simulink model "ctrl_HSMBObserver"  (R2015a)
settings: Solver=ode3  StartTime=0.0  StopTime=inf  FixedStep=0.01  RelTol=1e-3
values from neighbouring files (symbols this model uses):
  C = [C1;C2;C3;C4;C5;C6]    [initfile.m]    (also in thrustallocationQuadraticFixed.m)
  D = 3.0/100    (= 0.03)    [initfile.m]    (also in thrustallocationQuadraticFixed.m = 0.0411111111111)
  eps_c = 5    [initfile.m]
  epsilon = 0.5    [initfile.m]    (also in thrustallocationPseudo.m = u(10); thrustallocationQuadraticFixed.m = u(10))
  hd = c2d(H1,0.01,'foh')    [initfile.m]
  hd2 = c2d(H2,0.01,'zoh')    [initfile.m]
  I_s = 25000 /747225    (= 0.0334571246947)    [initfile.m]
  k_cc = 1    [initfile.m]
  K_omega = 0.3    [initfile.m]
  K_q1f = 0.0113    [initfile.m]
  K_q1r = K_q1f    (= 0.0113)    [initfile.m]
  K_q2f = 0.0117    [initfile.m]
  K_q2r = K_q2f    (= 0.0117)    [initfile.m]
  K_q3f = 0.0113    [initfile.m]
  K_q3r = K_q3f    (= 0.0113)    [initfile.m]
  K_q4f = 0.0169    [initfile.m]
  K_q4r = K_q4f    (= 0.0169)    [initfile.m]
  K_q5f = 0.0144    [initfile.m]
  K_q5r = K_q5f    (= 0.0144)    [initfile.m]
  K_q6f = 0.0168    [initfile.m]
  K_q6r = K_q6f    (= 0.0168)    [initfile.m]
  K_T1f = 0.3763    [initfile.m]
  K_T1r = K_T1f    (= 0.3763)    [initfile.m]
  K_T2f = 0.3901    [initfile.m]
  K_T2r = K_T2f    (= 0.3901)    [initfile.m]
  K_T3f = 0.3776    [initfile.m]
  K_T3r = K_T3f    (= 0.3776)    [initfile.m]
  K_T4f = 0.5641    [initfile.m]
  K_T4r = K_T4f    (= 0.5641)    [initfile.m]
  K_T5f = 0.4799    [initfile.m]
  K_T5r = K_T5f    (= 0.4799)    [initfile.m]
  K_T6f = 0.5588    [initfile.m]
  K_T6r = K_T6f    (= 0.5588)    [initfile.m]
  Kp = 3.3    [initfile.m]
  Max_Acceleration = 5    [initfile.m]
  Max_rotation = 12*sqrt(lambda)    [initfile.m]
  Max_thrust = 1.5    [initfile.m]
  Min_thrust = -0.8    [initfile.m]
  n_c = 5    [initfile.m]
  n_max = 152    [initfile.m]
  p_cc = 0.5    [initfile.m]
  pwm_thr1_backward = coeffvalues(ForceToPWM)    [initfile.m]
  pwm_thr1_forward = coeffvalues(ForceToPWM)    [initfile.m]
  pwm_thr2_backward = coeffvalues(ForceToPWM)    [initfile.m]
  pwm_thr2_forward = coeffvalues(ForceToPWM)    [initfile.m]
  pwm_thr3_backward = coeffvalues(ForceToPWM)    [initfile.m]
  pwm_thr3_forward = coeffvalues(ForceToPWM)    [initfile.m]
  pwm_thr4_backward = coeffvalues(ForceToPWM)    [initfile.m]
  pwm_thr4_forward = coeffvalues(ForceToPWM)    [initfile.m]
  pwm_thr5_backward = coeffvalues(ForceToPWM)    [initfile.m]
  pwm_thr5_forward = coeffvalues(ForceToPWM)    [initfile.m]
  pwm_thr6_backward = coeffvalues(ForceToPWM)    [initfile.m]
  pwm_thr6_forward = coeffvalues(ForceToPWM)    [initfile.m]
  Q_f0 = 0.3    [initfile.m]
  r_cc = 4    [initfile.m]
  Rho = Rho_m    (= 1000)    [initfile.m]
  ts = [-1 0]    [thrustallocationPseudo.m]    (also in thrustallocationQuadraticFixed.m)
undefined symbols (not defined in the file or in its folder): AFB, arm, Att, Control, Damping, FaultDet, Glob, Grip, IntActionType, Mass, NPO, Obs, Omg0_min, Q_max, ReferenceMdl, Sensor, Sim, SwLogic, tau, Thruster, Thruster_lock
libraries: dspmtrx3 x14, marine_gnc x11, simulink_extras x9, dspstat3 x9, simulink x9, dsparch4 x6, dspspect3 x6
(part 6 of 7)

== system ctrl_HSMBObserver/Thruster control /Thruster 6/Thruster control ==
  note: Q_ci
  note: Q_if
  note: Q_ff
  note: Q_ff0
  note: Q_ff1
  note: Friction compensation
  "T_d " : Inport
  n : Inport  Port=2
  Acceleration limiter : RateLimiter  RisingSlewLimit=Max_Acceleration  FallingSlewLimit=-Max_Acceleration  SampleTimeMode=inherited
  Constant1 : Constant  Value=hd.num{1,1}  VectorParams1D=off
  Constant2 : Constant  Value=hd.den{1,1}  VectorParams1D=off
  Controller chosen : MultiPortSwitch  Inputs=5
  Core controller : Subsystem
  Delay : Delay  DelayLength=1  InitialCondition=0
  Discrete Transfer Fcn : DiscreteTransferFcn  NumeratorSource=Input port  Numerator=[8.76e-05 0.0003481 8.648e-05]  DenominatorSource=Input port  Denominator=[1 -1.974 0.9746]  SampleTime=0.01  a0EqualsOne=on
      settings: InputPortMap=u0,p1,p3
  Discrete Derivative : simulink/Discrete/Discrete Derivative  gainval=1.0  ICPrevScaledInput=0.0  InputProcessing=Inherited  OutMin=[]  OutMax=[]  OutDataType=fixdt(1, 16)  OutScaling=2^-10  DoSatur=off
  Inertia compensation : Gain  Gain=I_s*2*pi
  MATLAB Function : MATLAB Function  TreatAsAtomicUnit=on
  Memory : Memory  X0=1
  NaN : Constant  Value=0
  Qf_0 : Gain  Gain=Q_f0
  Qff_0(nr) : Gain  Gain=epsilon/n_max
  Qff_1(nr) : Gain  Gain=K_omega*2*pi
  Sum : Sum  Inputs=+++
  Sum1 : Sum  Inputs=++|
  Supervisor : MATLAB Function  TreatAsAtomicUnit=on
  Trigonometric Function : Trigonometry  Operator=tanh
  Qc : Outport
  wires:
  Sum/1 -> Qc/1
  MATLAB Function/2(T_r) -> Core controller/2("Tr ")
  Discrete Derivative/1 -> Acceleration limiter/1
  Qff_0(nr)/1 -> Trigonometric Function/1
  Trigonometric Function/1 -> Qf_0/1
  Sum1/1 -> Sum/2
  Core controller/1(Q_cn) -> Controller chosen/2
  Core controller/4(Qcc) -> Controller chosen/5
  NaN/1 -> Controller chosen/6
  Memory/1 -> Supervisor/1(control), Controller chosen/1
  Qff_1(nr)/1 -> Sum1/2
  Qf_0/1 -> Sum1/1
  Controller chosen/1 -> Sum/3
  Inertia compensation/1 -> Sum/1
  Core controller/3(Qcp) -> Controller chosen/4
  Core controller/2(Qcq) -> Controller chosen/3
  [controller] -> Supervisor/2(input)
  "T_d "/1 -> MATLAB Function/1(Td)
  [Rho] -> MATLAB Function/4(rho)
  [D] -> MATLAB Function/5(D)
  [eps_c] -> MATLAB Function/6(eps_c)
  [n_c] -> MATLAB Function/7(n_c)
  Constant1/1 -> Discrete Transfer Fcn/2
  Constant2/1 -> Discrete Transfer Fcn/3
  MATLAB Function/1(n_d) -> Discrete Transfer Fcn/1
  n/1 -> Supervisor/3(n), Core controller/3("n ")
  Discrete Transfer Fcn/1 -> Discrete Derivative/1, Core controller/1(n_r), Delay/1, Qff_0(nr)/1, Qff_1(nr)/1
  Acceleration limiter/1 -> Inertia compensation/1
  Supervisor/1(u) -> Memory/1
  Delay/1 -> MATLAB Function/8(n_r)
  [Kt6r] -> MATLAB Function/3(K_t0r)
  [Kt6f] -> MATLAB Function/2(K_t0)

== system ctrl_HSMBObserver/To meters and radians, noise and sampling/Sensor noise models/Compass measurement noise module ==
  Band-Limited White Noise : simulink/Sources/Band-Limited White Noise  Cov=0.4*1e-12  Ts=0.01  seed=[23341]
  Bias compass : Constant  Value=0
  Sum : Sum  Inputs=+|+  SaturateOnIntegerOverflow=on
  Psi_noised : Outport
  wires:
  Sum/1 -> Psi_noised/1
  Band-Limited White Noise/1 -> Sum/2
  Bias compass/1 -> Sum/1

== system ctrl_HSMBObserver/To meters and radians, noise and sampling/Sensor noise models/Position (x,y) GPS measurement noise module ==
  note: Ionosphere
  note: Troposphere
  Band-Limited White Noise : simulink/Sources/Band-Limited White Noise  Cov=[1e-7 1e-7]  Ts=0.01  seed=[23341]
  Band-Limited White Noise1 Thermal effects : simulink/Sources/Band-Limited White Noise  Cov=[Sensor.GPS.Pow_thermal]  Ts=0.01  seed=[23341]
  Bias atmosphere : Constant  Value=[Sensor.GPS.Bias_atm]
  Sum : Sum  Inputs=+++  SaturateOnIntegerOverflow=on
  noised_pos (x.y) : Outport
  wires:
  Bias atmosphere/1 -> Sum/1
  Band-Limited White Noise1 Thermal effects/1 -> Sum/3
  Sum/1 -> noised_pos (x.y)/1
  Band-Limited White Noise/1 -> Sum/2

== system ctrl_HSMBObserver/Hybrid Controller/Controllers/Subsystem1/fault, update to q == 1 ==
  u_PD : Inport
  Action Port : ActionPort  ActionType=then
  u_PD_hold : Outport
  wires:
  u_PD/1 -> u_PD_hold/1

== system ctrl_HSMBObserver/Hybrid Controller/Controllers/Tau PD-control/GNC: "Transposed rotation matrix yaw: RTz_psi" ==
  note: GNC: "Transposed
      | rotation matrix yaw"
  psi : Inport
  eta_tilde : Inport  Port=2  PortDimensions=3
  Fcn : Fcn  Expr=cos(u(1))*u(2)+sin(u(1))*u(3)
  Fcn1 : Fcn  Expr=-sin(u(1))*u(2)+cos(u(1))*u(3)
  Fcn2 : Fcn  Expr=u(4)
  Mux2 : Mux  Inputs=2
  Mux3 : Mux  Inputs=3
  R_T*eta_tilde : Outport
  wires:
  Mux2/1 -> Fcn1/1, Fcn/1, Fcn2/1
  Fcn/1 -> Mux3/1  "x_dot"
  Fcn1/1 -> Mux3/2  "y_dot"
  Fcn2/1 -> Mux3/3  "psi_dot"
  Mux3/1 -> R_T*eta_tilde/1  "eta_dot"
  psi/1 -> Mux2/1
  eta_tilde/1 -> Mux2/2

== system ctrl_HSMBObserver/Hybrid Controller/Controllers/Tau integral action: Normal or AFF/GNC: "Transposed rotation matrix yaw: RTz_psi"3 ==
  note: GNC: "Transposed
      | rotation matrix yaw"
  psi : Inport
  int_NED : Inport  Port=2  PortDimensions=3
  Fcn : Fcn  Expr=cos(u(1))*u(2)+sin(u(1))*u(3)
  Fcn1 : Fcn  Expr=-sin(u(1))*u(2)+cos(u(1))*u(3)
  Fcn2 : Fcn  Expr=u(4)
  Mux2 : Mux  Inputs=2
  Mux3 : Mux  Inputs=3
  R_T*eta_tilde : Outport
  wires:
  Mux2/1 -> Fcn1/1, Fcn/1, Fcn2/1
  Fcn/1 -> Mux3/1  "x_dot"
  Fcn1/1 -> Mux3/2  "y_dot"
  Fcn2/1 -> Mux3/3  "psi_dot"
  Mux3/1 -> R_T*eta_tilde/1  "eta_dot"
  psi/1 -> Mux2/1
  int_NED/1 -> Mux2/2

== system ctrl_HSMBObserver/Hybrid Controller/Controllers/Tau integral action: Normal or AFF/R(psi)nu1 ==
  Nu : Inport
  psi : Inport  Port=2
  Demux : Demux  Outputs=3
  Mux : Mux  Inputs=3
  Mux1 : Mux  Inputs=3
  Row1 : Fcn  Expr=cos(u(3))*u(1)-sin(u(3))*u(2)
  Row2 : Fcn  Expr=sin(u(3))*u(1)+cos(u(3))*u(2)
  Eta : Outport
  wires:
  Demux/3 -> Mux1/3
  Nu/1 -> Demux/1
  psi/1 -> Mux/3
  Demux/1 -> Mux/1
  Demux/2 -> Mux/2
  Mux/1 -> Row1/1, Row2/1
  Mux1/1 -> Eta/1
  Row2/1 -> Mux1/2
  Row1/1 -> Mux1/1

== system ctrl_HSMBObserver/Hybrid Controller/Nonlinear observer, version implemented 04.26.2016/Hybridgains - kappa determination/Subsystem ==
  eta_f : Inport
  Demux : Demux  Outputs=3
  Dot Product : DotProduct  InputSameDT=on  OutDataTypeStr=Inherit: Inherit via internal rule
  Mux : Mux  Inputs=3
  Radians to Degrees : simulink_extras/Transformations/Radians to Degrees
  Transpose : Math  Operator=transpose  SaturateOnIntegerOverflow=on
  norm(eta_eta_f) : Outport
  wires:
  Dot Product/1 -> norm(eta_eta_f)/1
  Demux/3 -> Radians to Degrees/1
  Demux/1 -> Mux/1
  Demux/2 -> Mux/2
  Radians to Degrees/1 -> Mux/3
  Mux/1 -> Transpose/1, Dot Product/2
  Transpose/1 -> Dot Product/1
  eta_f/1 -> Demux/1

== system ctrl_HSMBObserver/Hybrid Controller/Peak Frequency FFT/CalmWater choose PID1/If Action Subsystem ==
  Action Port : ActionPort  ActionType=then
  Constant : Constant  Value=Omg0_min
  omega_p : Outport
  wires:
  Constant/1 -> omega_p/1

== system ctrl_HSMBObserver/Hybrid Controller/Peak Frequency FFT/CalmWater choose PID1/If Action Subsystem1 ==
  In1 : Inport
  Action Port : ActionPort  ActionType=else
  Out1 : Outport
  wires:
  In1/1 -> Out1/1

== system ctrl_HSMBObserver/Hybrid Controller/Peak Frequency FFT/estimate w_p/Spectral Analysis ==
  eta_6DOF : Inport
  Analog Filter Design{,1..5} (6 alike) : dsparch4/Analog Filter Design  method=Butterworth  filttype=Highpass  N=2  Wlo=Control.SA.pssbnd  Whi=80  Rp=2  Rs=40
  Demux : Demux  Outputs=6
  FFT : Subsystem
  w_p : Outport
  wires:
  eta_6DOF/1 -> Demux/1
  Demux/1 -> Analog Filter Design/1
  Analog Filter Design/1 -> FFT/1(surge)
  Analog Filter Design1/1 -> FFT/2(sway)
  Analog Filter Design2/1 -> FFT/3(heave)
  FFT/1(w_p) -> w_p/1
  Demux/3 -> Analog Filter Design2/1
  Demux/2 -> Analog Filter Design1/1
  Demux/5 -> Analog Filter Design3/1
  Demux/6 -> Analog Filter Design4/1
  Analog Filter Design3/1 -> FFT/5(pitch)
  Analog Filter Design4/1 -> FFT/6(yaw)
  Demux/4 -> Analog Filter Design5/1
  Analog Filter Design5/1 -> FFT/4(roll)

== system ctrl_HSMBObserver/Hybrid Controller/Switching logic/Desired yaw rate/Stay with the current controlller ==
  In1 : Inport
  Action Port : ActionPort  ActionType=else
  Out1 : Outport
  wires:
  In1/1 -> Out1/1

== system ctrl_HSMBObserver/Hybrid Controller/Switching logic/Desired yaw rate/Switch to grip ==
  Action Port : ActionPort  ActionType=then
  Constant : Constant  Value=2
  Out1 : Outport
  wires:
  Constant/1 -> Out1/1

== system ctrl_HSMBObserver/Hybrid Controller/Switching logic/Performance/Stay with the current controlller ==
  In1 : Inport
  Action Port : ActionPort  ActionType=else
  Out1 : Outport
  wires:
  In1/1 -> Out1/1

== system ctrl_HSMBObserver/Hybrid Controller/Switching logic/Performance/Switch to NPO ==
  Action Port : ActionPort  ActionType=then
  Constant : Constant
  Out1 : Outport
  wires:
  Constant/1 -> Out1/1

== system ctrl_HSMBObserver/Hybrid Controller/Switching logic/Performance/Switch to grip ==
  Action Port : ActionPort  ActionType=elseif
  Constant : Constant  Value=2
  Out1 : Outport
  wires:
  Constant/1 -> Out1/1

== system ctrl_HSMBObserver/Hybrid Controller/nPDF/Subsystem/R^TKdR ==
  eta : Inport
  nu : Inport  Port=2
  Kd : Inport  Port=3
  Create Diagonal Matrix3 : dspmtrx3/Create Diagonal Matrix
  Matrix Multiply3 : Product  Multiplication=Matrix(*)
  Rotation matrix in yaw 1 : marine_gnc/Models/ Kinematics/Rotation matrix in yaw 
  Selector : Selector  InputPortWidth=3  Indices=3
  Transposed rotation matrix in yaw1 : marine_gnc/Models/ Kinematics/Transposed rotation  matrix in yaw
  R^TKdR*nu : Outport
  wires:
  Selector/1 -> Rotation matrix in yaw 1/1, Transposed rotation matrix in yaw1/1
  eta/1 -> Selector/1
  nu/1 -> Rotation matrix in yaw 1/2
  Transposed rotation matrix in yaw1/1 -> R^TKdR*nu/1
  Rotation matrix in yaw 1/1 -> Matrix Multiply3/2
  Create Diagonal Matrix3/1 -> Matrix Multiply3/1
  Kd/1 -> Create Diagonal Matrix3/1
  Matrix Multiply3/1 -> Transposed rotation matrix in yaw1/2

== system ctrl_HSMBObserver/Hybrid Controller/nPDF/Subsystem/S(r)*nu ==
  nu : Inport
  Constant : Constant  Value=[0 -1 0;1 0 0;0 0 0]
  Product : Product  Multiplication=Matrix(*)
  Product1 : Product
  Selector1 : Selector  InputPortWidth=3  Indices=3
  S(r)*nu : Outport
  wires:
  Product/1 -> S(r)*nu/1
  Product1/1 -> Product/1
  nu/1 -> Product/2, Selector1/1
  Constant/1 -> Product1/2
  Selector1/1 -> Product1/1

== system ctrl_HSMBObserver/Thruster control /Thruster 1/Thruster control/Core controller ==
  note: Core controller: Shaft speed
  n_r : Inport
  "Tr " : Inport  Port=2
  "n " : Inport  Port=3
  Core controller: Torque,Power and Combined Torque/Power : MATLAB Function  TreatAsAtomicUnit=on
  Integrator : Integrator  ExternalReset=either  UpperSaturationLimit=Q_max  LowerSaturationLimit=-Q_max
  Ki : Gain  Gain=Kp/0.05
  Kp : Gain  Gain=Kp
  Sum : Sum  Inputs=+|-
  Sum1 : Sum  Inputs=|++
  reset : S-Function  Priority=1  FunctionName=NIVeriStandIO  Parameters=width dtype portnum stime stype btype  mask(NI VeriStand Inport){portnum=1, width=-1, stime=-1, dtype=auto, stype=auto, btype=1}
      mask prompts: portnum "Port number:"; width "Port dimensions (-1 for dynamically sized):"; stime "Sample time (-1 for inherited):"; dtype "Data type:"; stype "Signal type:"; btype "Block type:"
      mask help: Use this inport on any level of nested subsystems to allow NI VeriStand software to map signals to it.
      mask init:
      | NIVeriStandIO_init;
      settings: CopyFcn=NIVeriStand_MDL_functions('', 'IO_copy');  DeleteFcn=NIVeriStand_MDL_functions('', 'IO_delete');  MoveFcn=set_param(gcb, 'Mask', 'on');
      mask Callback portnum: NIVeriStand_MDL_functions('', 'IO_setportnum');
      mask TypeOptions dtype: auto | double | single | int8 | uint8 | int16 | uint16 | int32 | uint32 | boolean
      mask Callback dtype: NIVeriStand_MDL_functions('', 'IO_booleansignal');
      mask TypeOptions stype: auto | real | complex
      mask Display:
      | patch([-x x], [-y y], [.90980 .81960 .32156]);
      | plot([xrad -x x xrad], [yrad -y y yrad]);
      | fprintf('NI In%d', portnum);
  Q_cn : Outport
  Qcq : Outport  Port=2
  Qcp : Outport  Port=3
  Qcc : Outport  Port=4
  wires:
  [k_cc] -> Core controller: Torque,Power and Combined Torque/Power/1(k_cc)
  [p_cc] -> Core controller: Torque,Power and Combined Torque/Power/2(p_cc)
  [r_cc] -> Core controller: Torque,Power and Combined Torque/Power/3(r_cc)
  Core controller: Torque,Power and Combined Torque/Power/3(Qcc) -> Qcc/1
  [Kt1f] -> Core controller: Torque,Power and Combined Torque/Power/5(K_t0)
  [D] -> Core controller: Torque,Power and Combined Torque/Power/7(D)
  [Kq1f] -> Core controller: Torque,Power and Combined Torque/Power/6(K_q0)
  [Rho] -> Core controller: Torque,Power and Combined Torque/Power/9(rho)
  "n "/1 -> Sum/2, Core controller: Torque,Power and Combined Torque/Power/4(n)
  "Tr "/1 -> Core controller: Torque,Power and Combined Torque/Power/8(Tr)
  Core controller: Torque,Power and Combined Torque/Power/2(Qcp) -> Qcp/1
  Core controller: Torque,Power and Combined Torque/Power/1(Qcq) -> Qcq/1
  n_r/1 -> Sum/1
  Ki/1 -> Integrator/1
  Kp/1 -> Sum1/1
  Integrator/1 -> Sum1/2
  Sum1/1 -> Q_cn/1
  Sum/1 -> Ki/1, Kp/1
  reset/1 -> Integrator/2
  [eps_c] -> Core controller: Torque,Power and Combined Torque/Power/10(eps_c)
  [Kt1r] -> Core controller: Torque,Power and Combined Torque/Power/11(K_t0r)
  [Kq1r] -> Core controller: Torque,Power and Combined Torque/Power/12(K_q0r)

== system ctrl_HSMBObserver/Thruster control /Thruster 2/Thruster control/Core controller ==
  note: Core controller: Shaft speed
  n_r : Inport
  "Tr " : Inport  Port=2
  "n " : Inport  Port=3
  Core controller: Torque,Power and Combined Torque/Power : MATLAB Function  TreatAsAtomicUnit=on
  Integrator : Integrator  ExternalReset=either  UpperSaturationLimit=Q_max  LowerSaturationLimit=-Q_max
  Ki : Gain  Gain=Kp/0.05
  Kp : Gain  Gain=Kp
  Sum : Sum  Inputs=+|-
  Sum1 : Sum  Inputs=|++
  reset : S-Function  Priority=1  FunctionName=NIVeriStandIO  Parameters=width dtype portnum stime stype btype  mask(NI VeriStand Inport){portnum=1, width=-1, stime=-1, dtype=auto, stype=auto, btype=1}
      mask prompts: portnum "Port number:"; width "Port dimensions (-1 for dynamically sized):"; stime "Sample time (-1 for inherited):"; dtype "Data type:"; stype "Signal type:"; btype "Block type:"
      mask help: Use this inport on any level of nested subsystems to allow NI VeriStand software to map signals to it.
      mask init:
      | NIVeriStandIO_init;
      settings: CopyFcn=NIVeriStand_MDL_functions('', 'IO_copy');  DeleteFcn=NIVeriStand_MDL_functions('', 'IO_delete');  MoveFcn=set_param(gcb, 'Mask', 'on');
      mask Callback portnum: NIVeriStand_MDL_functions('', 'IO_setportnum');
      mask TypeOptions dtype: auto | double | single | int8 | uint8 | int16 | uint16 | int32 | uint32 | boolean
      mask Callback dtype: NIVeriStand_MDL_functions('', 'IO_booleansignal');
      mask TypeOptions stype: auto | real | complex
      mask Display:
      | patch([-x x], [-y y], [.90980 .81960 .32156]);
      | plot([xrad -x x xrad], [yrad -y y yrad]);
      | fprintf('NI In%d', portnum);
  Q_cn : Outport
  Qcq : Outport  Port=2
  Qcp : Outport  Port=3
  Qcc : Outport  Port=4
  wires:
  n_r/1 -> Sum/1
  Ki/1 -> Integrator/1
  Kp/1 -> Sum1/1
  Integrator/1 -> Sum1/2
  Sum/1 -> Ki/1, Kp/1
  Sum1/1 -> Q_cn/1
  reset/1 -> Integrator/2
  [k_cc] -> Core controller: Torque,Power and Combined Torque/Power/1(k_cc)
  [p_cc] -> Core controller: Torque,Power and Combined Torque/Power/2(p_cc)
  [r_cc] -> Core controller: Torque,Power and Combined Torque/Power/3(r_cc)
  Core controller: Torque,Power and Combined Torque/Power/3(Qcc) -> Qcc/1
  [Kt2f] -> Core controller: Torque,Power and Combined Torque/Power/5(K_t0)
  [D] -> Core controller: Torque,Power and Combined Torque/Power/7(D)
  [Kq2f] -> Core controller: Torque,Power and Combined Torque/Power/6(K_q0)
  [Rho] -> Core controller: Torque,Power and Combined Torque/Power/9(rho)
  "n "/1 -> Core controller: Torque,Power and Combined Torque/Power/4(n), Sum/2
  "Tr "/1 -> Core controller: Torque,Power and Combined Torque/Power/8(Tr)
  Core controller: Torque,Power and Combined Torque/Power/2(Qcp) -> Qcp/1
  Core controller: Torque,Power and Combined Torque/Power/1(Qcq) -> Qcq/1
  [eps_c] -> Core controller: Torque,Power and Combined Torque/Power/10(eps_c)
  [Kt2r] -> Core controller: Torque,Power and Combined Torque/Power/11(K_t0r)
  [Kq2r] -> Core controller: Torque,Power and Combined Torque/Power/12(K_q0r)

== system ctrl_HSMBObserver/Thruster control /Thruster 3/Thruster control/Core controller ==
  note: Core controller: Shaft speed
  n_r : Inport
  "Tr " : Inport  Port=2
  "n " : Inport  Port=3
  Core controller: Torque,Power and Combined Torque/Power : MATLAB Function  TreatAsAtomicUnit=on
  Integrator : Integrator  ExternalReset=either  UpperSaturationLimit=Q_max  LowerSaturationLimit=-Q_max
  Ki : Gain  Gain=Kp/0.05
  Kp : Gain  Gain=Kp
  Sum : Sum  Inputs=+|-
  Sum1 : Sum  Inputs=|++
  reset : S-Function  Priority=1  FunctionName=NIVeriStandIO  Parameters=width dtype portnum stime stype btype  mask(NI VeriStand Inport){portnum=1, width=-1, stime=-1, dtype=auto, stype=auto, btype=1}
      mask prompts: portnum "Port number:"; width "Port dimensions (-1 for dynamically sized):"; stime "Sample time (-1 for inherited):"; dtype "Data type:"; stype "Signal type:"; btype "Block type:"
      mask help: Use this inport on any level of nested subsystems to allow NI VeriStand software to map signals to it.
      mask init:
      | NIVeriStandIO_init;
      settings: CopyFcn=NIVeriStand_MDL_functions('', 'IO_copy');  DeleteFcn=NIVeriStand_MDL_functions('', 'IO_delete');  MoveFcn=set_param(gcb, 'Mask', 'on');
      mask Callback portnum: NIVeriStand_MDL_functions('', 'IO_setportnum');
      mask TypeOptions dtype: auto | double | single | int8 | uint8 | int16 | uint16 | int32 | uint32 | boolean
      mask Callback dtype: NIVeriStand_MDL_functions('', 'IO_booleansignal');
      mask TypeOptions stype: auto | real | complex
      mask Display:
      | patch([-x x], [-y y], [.90980 .81960 .32156]);
      | plot([xrad -x x xrad], [yrad -y y yrad]);
      | fprintf('NI In%d', portnum);
  Q_cn : Outport
  Qcq : Outport  Port=2
  Qcp : Outport  Port=3
  Qcc : Outport  Port=4
  wires:
  n_r/1 -> Sum/1
  Ki/1 -> Integrator/1
  Kp/1 -> Sum1/1
  Integrator/1 -> Sum1/2
  Sum/1 -> Ki/1, Kp/1
  Sum1/1 -> Q_cn/1
  reset/1 -> Integrator/2
  [k_cc] -> Core controller: Torque,Power and Combined Torque/Power/1(k_cc)
  [p_cc] -> Core controller: Torque,Power and Combined Torque/Power/2(p_cc)
  [r_cc] -> Core controller: Torque,Power and Combined Torque/Power/3(r_cc)
  Core controller: Torque,Power and Combined Torque/Power/3(Qcc) -> Qcc/1
  [Kt3f] -> Core controller: Torque,Power and Combined Torque/Power/5(K_t0)
  [D] -> Core controller: Torque,Power and Combined Torque/Power/7(D)
  [Kq3f] -> Core controller: Torque,Power and Combined Torque/Power/6(K_q0)
  [Rho] -> Core controller: Torque,Power and Combined Torque/Power/9(rho)
  "n "/1 -> Sum/2, Core controller: Torque,Power and Combined Torque/Power/4(n)
  "Tr "/1 -> Core controller: Torque,Power and Combined Torque/Power/8(Tr)
  Core controller: Torque,Power and Combined Torque/Power/2(Qcp) -> Qcp/1
  Core controller: Torque,Power and Combined Torque/Power/1(Qcq) -> Qcq/1
  [eps_c] -> Core controller: Torque,Power and Combined Torque/Power/10(eps_c)
  [Kt3r] -> Core controller: Torque,Power and Combined Torque/Power/11(K_t0r)
  [Kq3r] -> Core controller: Torque,Power and Combined Torque/Power/12(K_q0r)

== system ctrl_HSMBObserver/Thruster control /Thruster 4/Thruster control/Core controller ==
  note: Core controller: Shaft speed
  n_r : Inport
  "Tr " : Inport  Port=2
  "n " : Inport  Port=3
  Core controller: Torque,Power and Combined Torque/Power : MATLAB Function  TreatAsAtomicUnit=on
  Integrator : Integrator  ExternalReset=either  UpperSaturationLimit=Q_max  LowerSaturationLimit=-Q_max
  Ki : Gain  Gain=Kp/0.05
  Kp : Gain  Gain=Kp
  Sum : Sum  Inputs=+|-
  Sum1 : Sum  Inputs=|++
  reset : S-Function  Priority=1  FunctionName=NIVeriStandIO  Parameters=width dtype portnum stime stype btype  mask(NI VeriStand Inport){portnum=1, width=-1, stime=-1, dtype=auto, stype=auto, btype=1}
      mask prompts: portnum "Port number:"; width "Port dimensions (-1 for dynamically sized):"; stime "Sample time (-1 for inherited):"; dtype "Data type:"; stype "Signal type:"; btype "Block type:"
      mask help: Use this inport on any level of nested subsystems to allow NI VeriStand software to map signals to it.
      mask init:
      | NIVeriStandIO_init;
      settings: CopyFcn=NIVeriStand_MDL_functions('', 'IO_copy');  DeleteFcn=NIVeriStand_MDL_functions('', 'IO_delete');  MoveFcn=set_param(gcb, 'Mask', 'on');
      mask Callback portnum: NIVeriStand_MDL_functions('', 'IO_setportnum');
      mask TypeOptions dtype: auto | double | single | int8 | uint8 | int16 | uint16 | int32 | uint32 | boolean
      mask Callback dtype: NIVeriStand_MDL_functions('', 'IO_booleansignal');
      mask TypeOptions stype: auto | real | complex
      mask Display:
      | patch([-x x], [-y y], [.90980 .81960 .32156]);
      | plot([xrad -x x xrad], [yrad -y y yrad]);
      | fprintf('NI In%d', portnum);
  Q_cn : Outport
  Qcq : Outport  Port=2
  Qcp : Outport  Port=3
  Qcc : Outport  Port=4
  wires:
  n_r/1 -> Sum/1
  Ki/1 -> Integrator/1
  Kp/1 -> Sum1/1
  Integrator/1 -> Sum1/2
  Sum/1 -> Ki/1, Kp/1
  Sum1/1 -> Q_cn/1
  [k_cc] -> Core controller: Torque,Power and Combined Torque/Power/1(k_cc)
  [p_cc] -> Core controller: Torque,Power and Combined Torque/Power/2(p_cc)
  [r_cc] -> Core controller: Torque,Power and Combined Torque/Power/3(r_cc)
  Core controller: Torque,Power and Combined Torque/Power/3(Qcc) -> Qcc/1
  [Kt4f] -> Core controller: Torque,Power and Combined Torque/Power/5(K_t0)
  [D] -> Core controller: Torque,Power and Combined Torque/Power/7(D)
  [Kq4f] -> Core controller: Torque,Power and Combined Torque/Power/6(K_q0)
  [Rho] -> Core controller: Torque,Power and Combined Torque/Power/9(rho)
  "n "/1 -> Core controller: Torque,Power and Combined Torque/Power/4(n), Sum/2
  "Tr "/1 -> Core controller: Torque,Power and Combined Torque/Power/8(Tr)
  Core controller: Torque,Power and Combined Torque/Power/2(Qcp) -> Qcp/1
  Core controller: Torque,Power and Combined Torque/Power/1(Qcq) -> Qcq/1
  [eps_c] -> Core controller: Torque,Power and Combined Torque/Power/10(eps_c)
  [Kt4r] -> Core controller: Torque,Power and Combined Torque/Power/11(K_t0r)
  [Kq4r] -> Core controller: Torque,Power and Combined Torque/Power/12(K_q0r)
  reset/1 -> Integrator/2

== system ctrl_HSMBObserver/Thruster control /Thruster 5/Thruster control/Core controller ==
  note: Core controller: Shaft speed
  n_r : Inport
  "Tr " : Inport  Port=2
  "n " : Inport  Port=3
  Core controller: Torque,Power and Combined Torque/Power : MATLAB Function  TreatAsAtomicUnit=on
  Integrator : Integrator  ExternalReset=either  UpperSaturationLimit=Q_max  LowerSaturationLimit=-Q_max
  Ki : Gain  Gain=Kp/0.05
  Kp : Gain  Gain=Kp
  Sum : Sum  Inputs=+|-
  Sum1 : Sum  Inputs=|++
  reset : S-Function  Priority=1  FunctionName=NIVeriStandIO  Parameters=width dtype portnum stime stype btype  mask(NI VeriStand Inport){portnum=1, width=-1, stime=-1, dtype=auto, stype=auto, btype=1}
      mask prompts: portnum "Port number:"; width "Port dimensions (-1 for dynamically sized):"; stime "Sample time (-1 for inherited):"; dtype "Data type:"; stype "Signal type:"; btype "Block type:"
      mask help: Use this inport on any level of nested subsystems to allow NI VeriStand software to map signals to it.
      mask init:
      | NIVeriStandIO_init;
      settings: CopyFcn=NIVeriStand_MDL_functions('', 'IO_copy');  DeleteFcn=NIVeriStand_MDL_functions('', 'IO_delete');  MoveFcn=set_param(gcb, 'Mask', 'on');
      mask Callback portnum: NIVeriStand_MDL_functions('', 'IO_setportnum');
      mask TypeOptions dtype: auto | double | single | int8 | uint8 | int16 | uint16 | int32 | uint32 | boolean
      mask Callback dtype: NIVeriStand_MDL_functions('', 'IO_booleansignal');
      mask TypeOptions stype: auto | real | complex
      mask Display:
      | patch([-x x], [-y y], [.90980 .81960 .32156]);
      | plot([xrad -x x xrad], [yrad -y y yrad]);
      | fprintf('NI In%d', portnum);
  Q_cn : Outport
  Qcq : Outport  Port=2
  Qcp : Outport  Port=3
  Qcc : Outport  Port=4
  wires:
  n_r/1 -> Sum/1
  Ki/1 -> Integrator/1
  Kp/1 -> Sum1/1
  Integrator/1 -> Sum1/2
  Sum/1 -> Ki/1, Kp/1
  Sum1/1 -> Q_cn/1
  reset/1 -> Integrator/2
  [k_cc] -> Core controller: Torque,Power and Combined Torque/Power/1(k_cc)
  [p_cc] -> Core controller: Torque,Power and Combined Torque/Power/2(p_cc)
  [r_cc] -> Core controller: Torque,Power and Combined Torque/Power/3(r_cc)
  Core controller: Torque,Power and Combined Torque/Power/3(Qcc) -> Qcc/1
  [Kt5f] -> Core controller: Torque,Power and Combined Torque/Power/5(K_t0)
  [D] -> Core controller: Torque,Power and Combined Torque/Power/7(D)
  [Kq5f] -> Core controller: Torque,Power and Combined Torque/Power/6(K_q0)
  [Rho] -> Core controller: Torque,Power and Combined Torque/Power/9(rho)
  "n "/1 -> Core controller: Torque,Power and Combined Torque/Power/4(n), Sum/2
  "Tr "/1 -> Core controller: Torque,Power and Combined Torque/Power/8(Tr)
  Core controller: Torque,Power and Combined Torque/Power/2(Qcp) -> Qcp/1
  Core controller: Torque,Power and Combined Torque/Power/1(Qcq) -> Qcq/1
  [eps_c] -> Core controller: Torque,Power and Combined Torque/Power/10(eps_c)
  [Kt5r] -> Core controller: Torque,Power and Combined Torque/Power/11(K_t0r)
  [Kq5r] -> Core controller: Torque,Power and Combined Torque/Power/12(K_q0r)

== system ctrl_HSMBObserver/Thruster control /Thruster 6/Thruster control/Core controller ==
  note: Core controller: Shaft speed
  n_r : Inport
  "Tr " : Inport  Port=2
  "n " : Inport  Port=3
  Core controller: Torque,Power and Combined Torque/Power : MATLAB Function  TreatAsAtomicUnit=on
  Integrator : Integrator  ExternalReset=either  UpperSaturationLimit=Q_max  LowerSaturationLimit=-Q_max
  Ki : Gain  Gain=Kp/0.05
  Kp : Gain  Gain=Kp
  Sum : Sum  Inputs=+|-
  Sum1 : Sum  Inputs=|++
  reset : S-Function  Priority=1  FunctionName=NIVeriStandIO  Parameters=width dtype portnum stime stype btype  mask(NI VeriStand Inport){portnum=1, width=-1, stime=-1, dtype=auto, stype=auto, btype=1}
      mask prompts: portnum "Port number:"; width "Port dimensions (-1 for dynamically sized):"; stime "Sample time (-1 for inherited):"; dtype "Data type:"; stype "Signal type:"; btype "Block type:"
      mask help: Use this inport on any level of nested subsystems to allow NI VeriStand software to map signals to it.
      mask init:
      | NIVeriStandIO_init;
      settings: CopyFcn=NIVeriStand_MDL_functions('', 'IO_copy');  DeleteFcn=NIVeriStand_MDL_functions('', 'IO_delete');  MoveFcn=set_param(gcb, 'Mask', 'on');
      mask Callback portnum: NIVeriStand_MDL_functions('', 'IO_setportnum');
      mask TypeOptions dtype: auto | double | single | int8 | uint8 | int16 | uint16 | int32 | uint32 | boolean
      mask Callback dtype: NIVeriStand_MDL_functions('', 'IO_booleansignal');
      mask TypeOptions stype: auto | real | complex
      mask Display:
      | patch([-x x], [-y y], [.90980 .81960 .32156]);
      | plot([xrad -x x xrad], [yrad -y y yrad]);
      | fprintf('NI In%d', portnum);
  Q_cn : Outport
  Qcq : Outport  Port=2
  Qcp : Outport  Port=3
  Qcc : Outport  Port=4
  wires:
  n_r/1 -> Sum/1
  Ki/1 -> Integrator/1
  Kp/1 -> Sum1/1
  Integrator/1 -> Sum1/2
  Sum/1 -> Ki/1, Kp/1
  Sum1/1 -> Q_cn/1
  reset/1 -> Integrator/2
  [k_cc] -> Core controller: Torque,Power and Combined Torque/Power/1(k_cc)
  [p_cc] -> Core controller: Torque,Power and Combined Torque/Power/2(p_cc)
  [r_cc] -> Core controller: Torque,Power and Combined Torque/Power/3(r_cc)
  Core controller: Torque,Power and Combined Torque/Power/3(Qcc) -> Qcc/1
  [Kt6f] -> Core controller: Torque,Power and Combined Torque/Power/5(K_t0)
  [D] -> Core controller: Torque,Power and Combined Torque/Power/7(D)
  [Kq6f] -> Core controller: Torque,Power and Combined Torque/Power/6(K_q0)
  [Rho] -> Core controller: Torque,Power and Combined Torque/Power/9(rho)
  "n "/1 -> Core controller: Torque,Power and Combined Torque/Power/4(n), Sum/2
  "Tr "/1 -> Core controller: Torque,Power and Combined Torque/Power/8(Tr)
  Core controller: Torque,Power and Combined Torque/Power/2(Qcp) -> Qcp/1
  Core controller: Torque,Power and Combined Torque/Power/1(Qcq) -> Qcq/1
  [eps_c] -> Core controller: Torque,Power and Combined Torque/Power/10(eps_c)
  [Kt6r] -> Core controller: Torque,Power and Combined Torque/Power/11(K_t0r)
  [Kq6r] -> Core controller: Torque,Power and Combined Torque/Power/12(K_q0r)

== system ctrl_HSMBObserver/Hybrid Controller/Peak Frequency FFT/estimate w_p/Spectral Analysis/FFT ==
  surge : Inport
  sway : Inport  Port=2
  heave : Inport  Port=3
  roll : Inport  Port=4
  pitch : Inport  Port=5
  yaw : Inport  Port=6
  Hz_to_rad/s : Gain  Gain=2*pi  SaturateOnIntegerOverflow=on  OutDataTypeStr=Inherit: Same as input  ParamDataTypeStr=Inherit: Same as input
  Rate Transition : RateTransition  OutPortSampleTime=0.01
  "wave freq estimator using the Burg parametric/ max entropy method " : Subsystem  mask{Fs=Control.SA.SampleFreq, b1=Control.SA.BufferSize, nfft=Control.SA.FFTlength, burg_order=Control.SA.BurgOrder, ovl=Control.SA.Overlap}
      mask prompts: Fs "Sample frequency=Fs"; b1 "Size buffer 1=b1"; nfft "FFT length=nfft"; burg_order "Order of Burg estim=burg_order"; ovl "Overlap=ovl"
  w_p : Outport
  wires:
  "wave freq estimator using the Burg parametric/ max entropy method "/1(w0_hat) -> Hz_to_rad/s/1
  surge/1 -> "wave freq estimator using the Burg parametric/ max entropy method "/1(x_pos)
  sway/1 -> "wave freq estimator using the Burg parametric/ max entropy method "/2(y_pos)
  heave/1 -> "wave freq estimator using the Burg parametric/ max entropy method "/3(z_pos)
  Hz_to_rad/s/1 -> Rate Transition/1
  roll/1 -> "wave freq estimator using the Burg parametric/ max entropy method "/4(phi_pos)
  pitch/1 -> "wave freq estimator using the Burg parametric/ max entropy method "/5(theta_pos)
  yaw/1 -> "wave freq estimator using the Burg parametric/ max entropy method "/6(psi_pos)
  Rate Transition/1 -> w_p/1

== system ctrl_HSMBObserver/Hybrid Controller/Peak Frequency FFT/estimate w_p/Spectral Analysis/FFT/wave freq estimator using the Burg parametric// max entropy method  ==
  x_pos : Inport
  y_pos : Inport  Port=2
  z_pos : Inport  Port=3
  phi_pos : Inport  Port=4
  theta_pos : Inport  Port=5
  psi_pos : Inport  Port=6
  PSD estimation with Burg method : Subsystem
  Peak frequency estimation : Subsystem
  w0_hat : Outport
  wires:
  PSD estimation with Burg method/1(x_PSD) -> Peak frequency estimation/1(x_PSD)
  PSD estimation with Burg method/2(y_PSD) -> Peak frequency estimation/2(y_PSD)
  PSD estimation with Burg method/3(z_PSD) -> Peak frequency estimation/3(z_PSD)
  PSD estimation with Burg method/4(phi_PSD) -> Peak frequency estimation/4(phi_PSD)
  PSD estimation with Burg method/5(theta_PSD) -> Peak frequency estimation/5(theta_PSD)
  PSD estimation with Burg method/6(psi_PSD) -> Peak frequency estimation/6(psi_PSD)
  x_pos/1 -> PSD estimation with Burg method/1(x_pos)
  y_pos/1 -> PSD estimation with Burg method/2(y_pos)
  z_pos/1 -> PSD estimation with Burg method/3(z_pos)
  phi_pos/1 -> PSD estimation with Burg method/4(phi_pos)
  theta_pos/1 -> PSD estimation with Burg method/5(theta_pos)
  psi_pos/1 -> PSD estimation with Burg method/6(psi_pos)
  Peak frequency estimation/1(w0_hat) -> w0_hat/1

== system ctrl_HSMBObserver/Hybrid Controller/Peak Frequency FFT/estimate w_p/Spectral Analysis/FFT/wave freq estimator using the Burg parametric// max entropy method /PSD estimation with Burg method ==
  x_pos : Inport
  y_pos : Inport  Port=2
  z_pos : Inport  Port=3
  phi_pos : Inport  Port=4
  theta_pos : Inport  Port=5
  psi_pos : Inport  Port=6
  Buffer b1 ** : Buffer  N=b1  V=ovl  TreatMby1Signals=One channel
  Buffer b1 *** : Buffer  N=b1  V=ovl  TreatMby1Signals=One channel
  Buffer b1 **** : Buffer  N=b1  V=ovl  TreatMby1Signals=One channel
  Buffer b1 ***1 : Buffer  N=b1  V=ovl  TreatMby1Signals=One channel
  Buffer b1 ***2 : Buffer  N=b1  V=ovl  TreatMby1Signals=One channel
  Buffer b1 **1 : Buffer  N=b1  V=ovl  TreatMby1Signals=One channel
  Burg Method{,1..5} (6 alike) : dspspect3/Burg Method  inheritOrd=off  ord=burg_order  inheritFFT=off  fftsize=nfft  inheritTs=on  Ts=1
  Zero-Order Hold{1..6} (6 alike) : ZeroOrderHold  SampleTime=1/Fs
  x_PSD : Outport
  y_PSD : Outport  Port=2
  z_PSD : Outport  Port=3
  phi_PSD : Outport  Port=4
  theta_PSD : Outport  Port=5
  psi_PSD : Outport  Port=6
  wires:
  x_pos/1 -> Zero-Order Hold1/1
  y_pos/1 -> Zero-Order Hold2/1
  z_pos/1 -> Zero-Order Hold3/1
  Zero-Order Hold1/1 -> Buffer b1 ****/1
  Zero-Order Hold2/1 -> Buffer b1 ***/1
  Zero-Order Hold3/1 -> Buffer b1 **/1
  theta_pos/1 -> Zero-Order Hold4/1
  psi_pos/1 -> Zero-Order Hold5/1
  Zero-Order Hold4/1 -> Buffer b1 ***1/1
  Zero-Order Hold5/1 -> Buffer b1 **1/1
  phi_pos/1 -> Zero-Order Hold6/1
  Zero-Order Hold6/1 -> Buffer b1 ***2/1
  Burg Method1/1 -> y_PSD/1
  Burg Method/1 -> x_PSD/1
  Burg Method2/1 -> z_PSD/1
  Buffer b1 **/1 -> Burg Method2/1
  Burg Method3/1 -> theta_PSD/1
  Burg Method4/1 -> psi_PSD/1
  Buffer b1 ***1/1 -> Burg Method3/1
  Buffer b1 **1/1 -> Burg Method4/1
  Burg Method5/1 -> phi_PSD/1
  Buffer b1 ***2/1 -> Burg Method5/1
  Buffer b1 ***/1 -> Burg Method1/1
  Buffer b1 ****/1 -> Burg Method/1

== system ctrl_HSMBObserver/Hybrid Controller/Peak Frequency FFT/estimate w_p/Spectral Analysis/FFT/wave freq estimator using the Burg parametric// max entropy method /Peak frequency estimation ==
  x_PSD : Inport
  y_PSD : Inport  Port=2
  z_PSD : Inport  Port=3
  phi_PSD : Inport  Port=4
  theta_PSD : Inport  Port=5
  psi_PSD : Inport  Port=6
  Demux : Demux  Outputs=6
  Fs/Nfft equally spaced frequencies : Gain  Gain=Fs/nfft  SaturateOnIntegerOverflow=on  OutDataTypeStr=Inherit: Same as input  ParamDataTypeStr=Inherit: Same as input
  Maximum{1..6} (6 alike) : dspstat3/Maximum  fcn=Index  reset=None  InputProcessing=Columns as channels (frame based)  indexBase=One  operateOver=Each column  Dimension=1  colComp=on  operation=maximum  roiEnable=off  roiType=Rectangles  roiPortion=Entire ROI  roiOutput=Individual statistics for each ROI  roiFlag=off  accumDataTypeStr=Inherit: Same as product output  accumLastDataTypeStr=Inherit: Same as product output  roundingMode=Floor  overflowMode=off
  Median : dspstat3/Median  sortAlg=Quick sort  directionMode=Each column  dimension=1  treatSBRowAsCol=on  outputDataTypeStr=Inherit: Same as accumulator  outputLastDataTypeStr=Inherit: Same as accumulator  outputMin=[]  outputMax=[]  accumDataTypeStr=Inherit: Same as product output  accumLastDataTypeStr=Inherit: Same as product output  roundingMode=Floor  overflowMode=off
      settings: allowOverrides=off
  Mux : Mux  Inputs=6
  Mux1 : Mux  Inputs=2
  Terminator{,1..6} (7 alike) : Terminator
  w0_hat : Outport
  wires:
  x_PSD/1 -> Maximum3/1
  y_PSD/1 -> Maximum1/1
  z_PSD/1 -> Maximum2/1
  Maximum3/1 -> Mux/1
  Maximum1/1 -> Mux/2
  Maximum2/1 -> Mux/3
  Mux/1 -> Fs/Nfft equally spaced frequencies/1  "max_index"
  psi_PSD/1 -> Maximum6/1
  theta_PSD/1 -> Maximum5/1
  phi_PSD/1 -> Maximum4/1
  Maximum4/1 -> Mux/4
  Maximum5/1 -> Mux/5
  Maximum6/1 -> Mux/6
  Fs/Nfft equally spaced frequencies/1 -> Demux/1  "w_null vector"
  Demux/1 -> Terminator1/1
  Demux/3 -> Terminator3/1, Mux1/1
  Demux/4 -> Terminator4/1
  Demux/5 -> Mux1/2, Terminator5/1
  Demux/6 -> Terminator6/1
  Median/1 -> w0_hat/1, Terminator/1
  Demux/2 -> Terminator2/1
  Mux1/1 -> Median/1

== matlab function ctrl_HSMBObserver/Hybrid Controller/Controllers/Tau PD-control/Ki eta_tilde1 ==
  data: nu_tilde input; tau_d output; Kd input
function tau_d = fcn(nu_tilde, Kd)


tau_d = Kd*nu_tilde;

== matlab function ctrl_HSMBObserver/Hybrid Controller/Controllers/Tau PD-control/MATLAB Function ==
  data: Kpin input; Kp output; t input; sf input
function Kp = fcn(Kpin,t,sf)
%#codegen

    Kp = Kpin*sf;

== matlab function ctrl_HSMBObserver/Hybrid Controller/Controllers/Tau PD-control/Ki eta_tilde ==
  data: eta_tilde_body input; tau_p output; Kp input
function tau_p = fcn(eta_tilde_body, Kp)


tau_p = Kp*eta_tilde_body;

== matlab function ctrl_HSMBObserver/Thruster control /Thrust and Shaft speed mapped to PWM/MATLAB Function1 ==
  data: Tc_in1 input; signal input; Tc_out output; Tc_in2 input
function Tc_out = fcn(Tc_in1,signal,Tc_in2)
%#codegen

if signal >= 0
    Tc_out = Tc_in1;
else %signal < 0
    Tc_out = Tc_in2;
end

== matlab function ctrl_HSMBObserver/TA fixed thrusters, pseudoinverse/MATLAB Function ==
  data: tau_c input; u output; ThrusterPosX input; ThrusterPosY input; alpha input
function u = fcn(tau_c,ThrusterPosX,ThrusterPosY,alpha)
% Pseudoinverse thrust allocation for fixed angles

% no thruster-thruster interaction
K = ones(1,6);

% Thruster configuration matrix
n_t = length(ThrusterPosX); % number of thrusters
B_surge = zeros(n_t,1); % Shells for faster computing
B_sway = zeros(n_t,1);  % Shells for faster computing
B_yaw = zeros(n_t,1);   % Shells for faster computing

for i = 1:1:n_t
  B_surge(i) = cosd(alpha(i));     %Thrust in x-direction for cartesian
  B_sway(i) = sind(alpha(i));      %Thrust in y-direction for cartesian
  B_yaw(i) = (sind(alpha(i))*ThrusterPosX(i) - cosd(alpha(i))*ThrusterPosY(i));
end

B = [B_surge,B_sway,B_yaw]';
B = B*diag(K); 

% pseudoinverse
% Bpinv = pinv(B);
Bpinv = [-0.3750    0.1251    0.0027;
   -0.1752   -0.1818   -0.2340;
   -0.1276    0.3831    0.3771;
    0.3750   -0.1251   -0.0027;
    0.1783    0.1719   -0.2263;
    0.1223   -0.3668    0.3825];    

u = Bpinv*tau_c;

== matlab function ctrl_HSMBObserver/Thruster control /Thruster 1/Propeller Hydrodynamics/Actual Force and Torque ==
  data: Ta output; n input; Qa output; Kq input; Kt input; Ktr input; Kqr input; Rho input; D input; eps_c input; env input; Pa output
function [Ta,Qa,Pa]= ActualForces(n,Kq,Kt,Ktr,Kqr,Rho,D,eps_c,env)
%#codegen
lambda_c = 0.5+0.5*tanh(eps_c*n/5); % Smooth switching between positive and negative thrust. 5 makes switch happen between -5 and 5
K_TC = Kt*lambda_c+(1-lambda_c)*Ktr;
K_QC = Kq*lambda_c+(1-lambda_c)*Kqr;

Ta = sign(n)*K_TC*Rho*(D^4)*n^2-env;
Qa = sign(n)*K_QC*Rho*(D^5)*n^2-env;
Pa = 2*pi*n*Qa;

== matlab function ctrl_HSMBObserver/Thruster control /Thruster 1/Thruster control/MATLAB Function ==
  data: Td input; n_d output; K_t0 input; K_t0r input; rho input; D input; eps_c input; n_c input; n_r input; T_r output
function [n_d,T_r]  = ReferenceGenerator(Td,K_t0,K_t0r,rho,D,eps_c,n_c,n_r)
%#codegen


n_d = sign(Td)*sqrt((abs(Td))/(rho*D^4*K_t0));

lambda_c = 0.5+0.5*tanh(eps_c*n_d/5); % Smooth switching between positive and negative thrust. 5 makes switch happen between -5 and 5
K_TC = K_t0*lambda_c+(1-lambda_c)*K_t0r;

T_r = sign(n_r)*K_TC*rho*D^4*n_r^2;

== matlab function ctrl_HSMBObserver/Thruster control /Thruster 1/Thruster control/Supervisor ==
  data: control input; input input; n input; u output
function u = fcn(control,input,n)
u = 1;
if control == 1
if input == 1
    u = 1;
elseif input == 2
    u = 2;
elseif input == 3 && n > 0 || input == 3 && n < 0
    u = 3;
elseif input == 4 || input == 3 && n == 0
    u = 4;
else 
    u = 5;
end
end

if control == 2
if input == 1
    u = 1;
elseif input == 2
    u = 2;
elseif input == 3 && n > 0 || input == 3 && n < 0
    u = 3;
elseif input == 4 || input == 3 && n == 0
    u = 4;
else 
    u = 5;
end
end

if control == 3
if input == 1
    u = 1;
elseif input == 2
    u = 2;
elseif input == 3 && n > 0 || input == 3 && n < 0
    u = 3;
elseif input == 4 || input == 3 && n == 0
    u = 4;
else 
    u = 5;
end
end

if control == 4
if input == 1
    u = 1;
elseif input == 2
    u = 2;
elseif input == 3 && n > 0 || input == 3 && n < 0
    u = 3;
elseif input == 4 || input == 3 && n == 0
    u = 4;
else 
    u = 5;
end
end

if control == 5
if input == 1
    u = 1;
elseif input == 2
    u = 2;
elseif input == 3 && n > 0 || input == 3 && n < 0
    u = 3;
elseif input == 4 || input == 3 && n == 0
    u = 4;
else 
    u = 5;
end
end

== matlab function ctrl_HSMBObserver/Thruster control /Thruster 1/Thruster control/Core controller/Core controller: Torque,Power and Combined Torque//Power ==
  data: Qcq output; Qcp output; k_cc input; p_cc input; r_cc input; n input; Qcc output; K_t0 input; K_q0 input; D input; Tr input; rho input; eps_c input; K_t0r input; K_q0r input
function [Qcq,Qcp,Qcc]= CoreControl(k_cc,p_cc,r_cc,n,K_t0,K_q0,D,Tr,rho,eps_c,K_t0r,K_q0r)
%#codegen

lambda_c = 0.5+0.5*tanh(eps_c*n/5);
K_TC = K_t0*lambda_c+(1-lambda_c)*K_t0r;
K_QC = K_q0*lambda_c+(1-lambda_c)*K_q0r;
Qcq = (K_QC/K_TC)*D*Tr;
if n == 0
    Qcp = 0;
else
Qcp = sign(Tr)*K_QC*(abs(Tr)^(3/2))/(sqrt(rho)*D*K_TC^(3/2)*abs(n));
end
alpha_c = exp(-k_cc*abs(p_cc*n)^r_cc);

Qcc = alpha_c*Qcq + (1-alpha_c)*Qcp;

== matlab function ctrl_HSMBObserver/Thruster control /Thrust and Shaft speed mapped to PWM/MATLAB Function2 ==
  data: Tc_in1 input; signal input; Tc_out output; Tc_in2 input
function Tc_out = fcn(Tc_in1,signal,Tc_in2)
%#codegen

if signal >= 0
    Tc_out = Tc_in1;
else %signal < 0
    Tc_out = Tc_in2;
end

== matlab function ctrl_HSMBObserver/Thruster control /Thruster 2/Propeller Hydrodynamics/Actual Force and Torque ==
  data: Ta output; n input; Qa output; Kq input; Kt input; Ktr input; Kqr input; Rho input; D input; eps_c input; env input
function [Ta,Qa]= ActualForces(n,Kq,Kt,Ktr,Kqr,Rho,D,eps_c,env)
%#codegen
lambda_c = 0.5+0.5*tanh(eps_c*n/5); % Smooth switching between positive and negative thrust. 5 makes switch happen between -5 and 5
K_TC = Kt*lambda_c+(1-lambda_c)*Ktr;
K_QC = Kq*lambda_c+(1-lambda_c)*Kqr;

Ta = sign(n)*K_TC*Rho*(D^4)*n^2-env;
Qa = sign(n)*K_QC*Rho*(D^5)*n^2-env;

== matlab function ctrl_HSMBObserver/Finding commanded forces in: [Surge,Sway,Yaw] ==
  data: thrust_actual input; commanded_tau output; alpha_actual input; PosX input; PosY input
function commanded_tau   = fcn(thrust_actual,alpha_actual,PosX,PosY)
%#codegen

Alpha_surge =[cosd(alpha_actual(1)) cosd(alpha_actual(2)) cosd(alpha_actual(3)) cosd(alpha_actual(4)) cosd(alpha_actual(5)) cosd(alpha_actual(6))];  
Alpha_sway = [sind(alpha_actual(1)) sind(alpha_actual(2)) sind(alpha_actual(3)) sind(alpha_actual(4)) sind(alpha_actual(5)) sind(alpha_actual(6))];
Alpha_yaw = [sind(alpha_actual(1))*PosX(1)-cosd(alpha_actual(1))*PosY(1) sind(alpha_actual(2))*PosX(2)-cosd(alpha_actual(2))*PosY(2) ...
             sind(alpha_actual(3))*PosX(3)-cosd(alpha_actual(3))*PosY(3) sind(alpha_actual(4))*PosX(4)-cosd(alpha_actual(4))*PosY(4) ...
             sind(alpha_actual(5))*PosX(5)-cosd(alpha_actual(5))*PosY(5) sind(alpha_actual(6))*PosX(6)-cosd(alpha_actual(6))*PosY(6)];

commanded_tau = [Alpha_surge;Alpha_sway;Alpha_yaw]*thrust_actual;

== matlab function ctrl_HSMBObserver/Hybrid Controller/Controllers/Tau PD-control/MATLAB Function1 ==
  data: Kdin input; Kd output; t input; sf input
function Kd = fcn(Kdin,t,sf)
%#codegen
    Kd = Kdin*sf;

== matlab function ctrl_HSMBObserver/Hybrid Controller/Controllers/Tau integral action: Normal or AFF/MATLAB Function ==
  data: IntActionType input; L1_in input; L2_in input; A_T_in input; beta_c_in input; q input; L1 output; L2 output; A_T output; beta_c output
function [L1,L2,A_T,beta_c] = fcn(IntActionType,L1_in,L2_in,A_T_in,beta_c_in,q)
% select integral action based on the value of q
% 
% 


% q = 1: Model based observer: should set AFF = 0, and L2 = 0
% q = 2: Signal based observer

if q == 1 
    L1 = L1_in;
    L2 = [0;0;0];
    A_T = A_T_in;
    beta_c = [0;0;0];
    
else
    L1 = L1_in;
    L2 = L2_in;
    A_T = A_T_in;
    beta_c = beta_c_in;
end

== matlab function ctrl_HSMBObserver/Thruster control /Thrust and Shaft speed mapped to PWM/MATLAB Function3 ==
  data: Tc_in1 input; signal input; Tc_out output; Tc_in2 input
function Tc_out = fcn(Tc_in1,signal,Tc_in2)
%#codegen

if signal >= 0
    Tc_out = Tc_in1;
else %signal < 0
    Tc_out = Tc_in2;
end

== matlab function ctrl_HSMBObserver/Thruster control /Thruster 2/Thruster control/Core controller/Core controller: Torque,Power and Combined Torque//Power ==
  data: Qcq output; Qcp output; k_cc input; p_cc input; r_cc input; n input; Qcc output; K_t0 input; K_q0 input; D input; Tr input; rho input; eps_c input; K_t0r input; K_q0r input
function [Qcq,Qcp,Qcc]= CoreControl(k_cc,p_cc,r_cc,n,K_t0,K_q0,D,Tr,rho,eps_c,K_t0r,K_q0r)
%#codegen

lambda_c = 0.5+0.5*tanh(eps_c*n/5);
K_TC = K_t0*lambda_c+(1-lambda_c)*K_t0r;
K_QC = K_q0*lambda_c+(1-lambda_c)*K_q0r;
Qcq = (K_QC/K_TC)*D*Tr;
if n == 0
    Qcp = 0;
else
Qcp = sign(Tr)*K_QC*(abs(Tr)^(3/2))/(sqrt(rho)*D*K_TC^(3/2)*abs(n));
end
alpha_c = exp(-k_cc*abs(p_cc*n)^r_cc);

Qcc = alpha_c*Qcq + (1-alpha_c)*Qcp;

== matlab function ctrl_HSMBObserver/Thruster control /Thruster 2/Thruster control/MATLAB Function ==
  data: Td input; n_d output; K_t0 input; K_t0r input; rho input; D input; eps_c input; n_c input; n_r input; T_r output
function [n_d,T_r]  = ReferenceGenerator(Td,K_t0,K_t0r,rho,D,eps_c,n_c,n_r)
%#codegen


n_d = sign(Td)*sqrt((abs(Td))/(rho*D^4*K_t0));

lambda_c = 0.5+0.5*tanh(eps_c*n_d/5); % Smooth switching between positive and negative thrust
K_TC = K_t0*lambda_c+(1-lambda_c)*K_t0r;

T_r = sign(n_r)*K_TC*rho*D^4*n_r^2;
